simulink model "Root_Locus"  (R2024a)
settings: Solver=VariableStepAuto  StartTime=0.0  StopTime=1200  RelTol=1e-3
model workspace (MAT data in the model file):
  At = 0.01309
libraries: simulink x2
settings Model: Creator=adamk  LastModifiedBy=krish

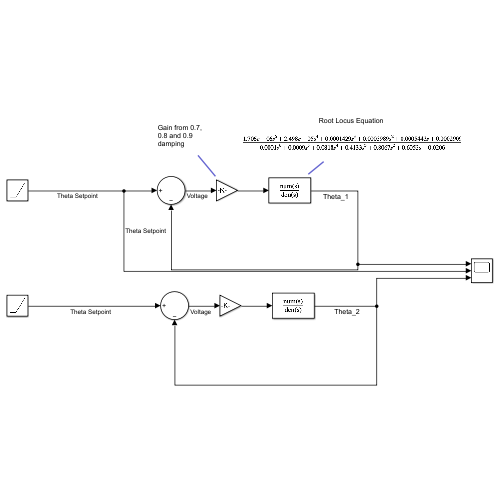
[thumbnail: Simulink's stored preview of the top-level diagram]
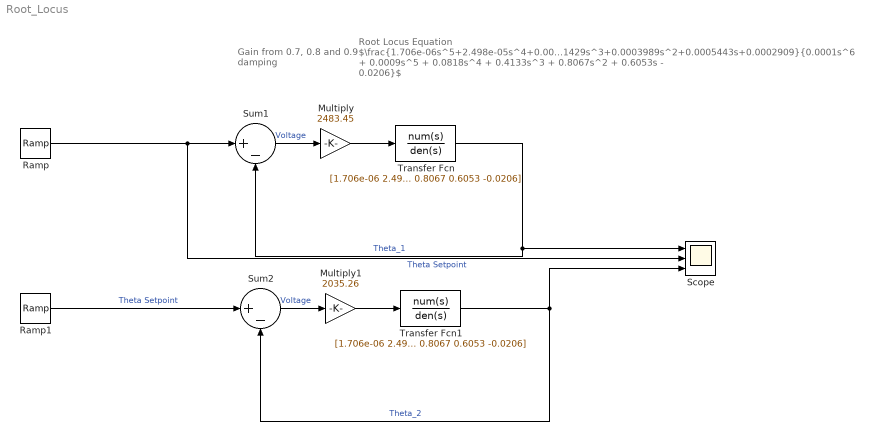
== system Root_Locus ==
  note: Root Locus Equation
      |
      | $\frac{1.706e-06s^5+2.498e-05s^4+0.0001429s^3+0.0003989s^2+0.0005443s+0.0002909}{0.0001s^6 + 0.0009s^5 + 0.0818s^4 + 0.4133s^3 + 0.8067s^2 + 0.6053s - 0.0206}$
  note: Gain from 0.7, 0.8 and 0.9 damping
  Multiply : Gain  Gain=2483.45
  Multiply1 : Gain  Gain=2035.26
  Ramp : simulink/Sources/Ramp  slope=1.333e-3  start=0  InitialOutput=0
  Ramp1 : simulink/Sources/Ramp  slope=1.333e-3  start=0  InitialOutput=0
  Scope : Scope  NumInputPorts=3
  Sum1 : Sum  Inputs=|+-
  Sum2 : Sum  Inputs=|+-
  Transfer Fcn : TransferFcn  Numerator=[1.706e-06 2.498e-05 0.0001429 0.0003989 0.0005443 0.0002909]  Denominator=[0.0001 0.0009 0.0818 0.4133 0.8067 0.6053 -0.0206]
  Transfer Fcn1 : TransferFcn  Numerator=[1.706e-06 2.498e-05 0.0001429 0.0003989 0.0005443 0.0002909]  Denominator=[0.0001 0.0009 0.0818 0.4133 0.8067 0.6053 -0.0206]
  wires:
  Transfer Fcn/1 -> Scope/1, Sum1/2  "Theta_1"
  Ramp/1 -> Scope/2, Sum1/1  "Theta Setpoint"
  Sum1/1 -> Multiply/1  "Voltage"
  Multiply/1 -> Transfer Fcn/1
  Multiply1/1 -> Transfer Fcn1/1
  Ramp1/1 -> Sum2/1  "Theta Setpoint"
  Sum2/1 -> Multiply1/1  "Voltage"
  Transfer Fcn1/1 -> Scope/3, Sum2/2  "Theta_2"
